simulink model "Adams_HW_Dynamic"  (R2023b)
settings: Solver=VariableStepAuto  StartTime=0.0  StopTime=10.0  RelTol=1e-3
values from neighbouring files (symbols this model uses):
  ddQ1 = x(7)    [Adams_HW1.m]    (also in BSM.m; Correct_new_data.m; MechanicalMechanics_Dynamic.m; MechanicalMechanics_Dynamic_adaptive_BSM.m)
  L1 = x(1)    [Adams_HW1.m]    (also in Adams_HW_DrawGIF.m = current_x(1); Adams_HW_DrawGIF_Y.m = current_x(1); BSM.m; Correct_new_data.m)
  L2 = x(2)    [Adams_HW1.m]    (also in Adams_HW_DrawGIF.m = current_x(2); Adams_HW_DrawGIF_Y.m = current_x(2); BSM.m; Correct_new_data.m)
  L3 = x(3)    [Adams_HW1.m]    (also in Adams_HW_DrawGIF.m = current_x(3); Adams_HW_DrawGIF_Y.m = current_x(3); BSM.m; Correct_new_data.m)
  L4 = x(4)    [Adams_HW1.m]    (also in Adams_HW_DrawGIF.m = current_x(4); Adams_HW_DrawGIF_Y.m = current_x(4); BSM.m; Correct_new_data.m)
  Q1 = x(5)    [Adams_HW1.m]    (also in Adams_HW_DrawGIF.m = current_x(5); Adams_HW_DrawGIF_Y.m = current_x(5); BSM.m; Correct_new_data.m)
  Q2 = Inition(1)    [Adams_HW1.m]    (also in BSM.m = x(8); Correct_new_data.m = x(8); GenerateSimplifiedMechanism.m = x(8); MechanicalMechanics_Dynamic.m = x(8))
  Q3 = x(11)    [Adams_HW1.m]    (also in Adams_HW_DrawGIF.m = current_x(11); Adams_HW_DrawGIF_Y.m = current_x(7); BSM.m; Correct_new_data.m)
settings Model: Creator=Akko  LastModifiedBy=Akko

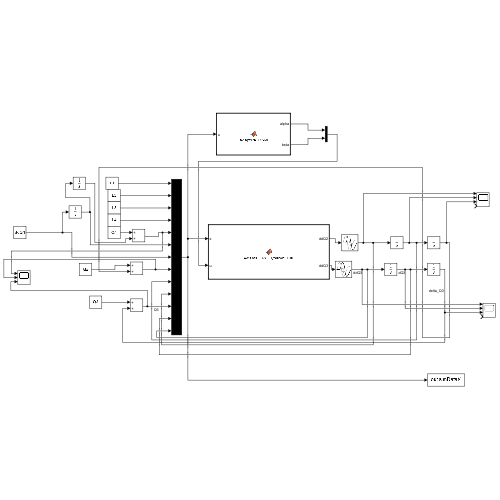
[thumbnail: Simulink's stored preview of the top-level diagram]
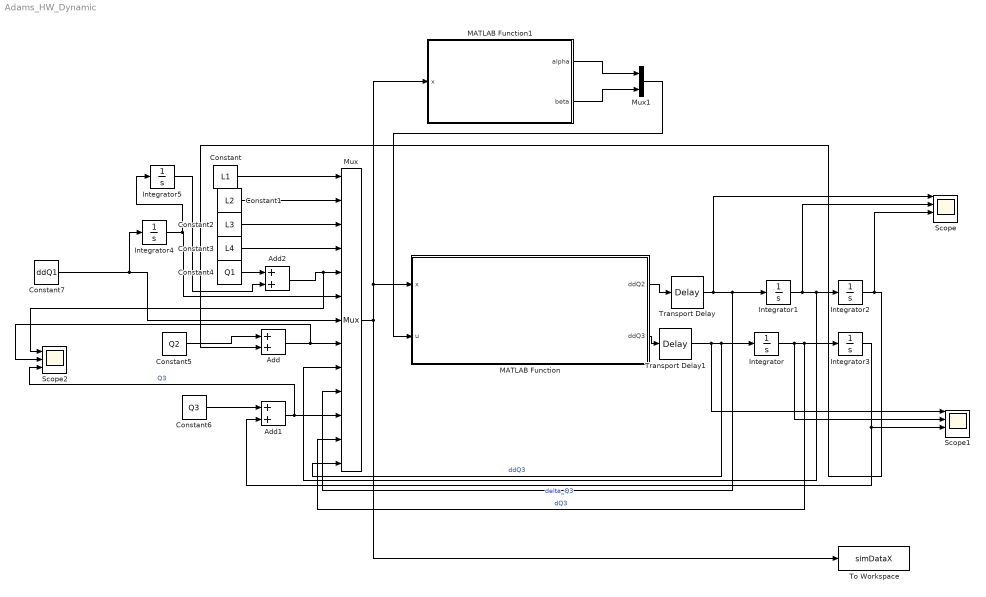
== system Adams_HW_Dynamic ==
  Add : Sum
  Add1 : Sum
  Add2 : Sum
  Constant : Constant  Value=L1
  Constant1 : Constant  Value=L2
  Constant2 : Constant  Value=L3
  Constant3 : Constant  Value=L4
  Constant4 : Constant  Value=Q1
  Constant5 : Constant  Value=Q2
  Constant6 : Constant  Value=Q3
  Constant7 : Constant  Value=ddQ1
  Integrator{,1..5} (6 alike) : Integrator
  MATLAB Function : MATLAB Function  TreatAsAtomicUnit=on
  MATLAB Function1 : MATLAB Function  TreatAsAtomicUnit=on
  Mux : Mux  Inputs=13
  Mux1 : Mux  Inputs=2
  Scope : Scope  NumInputPorts=4
  Scope1 : Scope  NumInputPorts=4
  Scope2 : Scope  NumInputPorts=3
  To Workspace : ToWorkspace  VariableName=simDataX  SampleTime=-1
  Transport Delay : TransportDelay  DelayTime=1e-4
  Transport Delay1 : TransportDelay  DelayTime=1e-4
  wires:
  Mux/1 -> MATLAB Function1/1("x "), MATLAB Function/1(x), To Workspace/1
  Constant/1 -> Mux/1
  Constant1/1 -> Mux/2
  Constant2/1 -> Mux/3
  Constant3/1 -> Mux/4
  MATLAB Function/2(ddQ3) -> Transport Delay1/1
  MATLAB Function/1(ddQ2) -> Transport Delay/1
  Transport Delay1/1 -> Scope1/1, Mux/13, Integrator/1  "ddQ3"
  Transport Delay/1 -> Scope/1, Mux/10, Integrator1/1
  Integrator1/1 -> Scope/2, Mux/9, Integrator2/1
  Integrator/1 -> Scope1/2, Mux/12, Integrator3/1  "dQ3"
  Integrator2/1 -> Scope/3, Add/2
  Constant5/1 -> Add/1
  Add/1 -> Scope2/2, Mux/8
  Add1/1 -> Mux/11, Scope2/3  "Q3"
  Constant6/1 -> Add1/1
  Integrator3/1 -> Scope1/3, Add1/2  "delta_Q3"
  Constant7/1 -> Integrator4/1, Mux/7
  Integrator4/1 -> Integrator5/1, Mux/6
  Add2/1 -> Scope2/1, Mux/5
  Constant4/1 -> Add2/1
  Integrator5/1 -> Add2/2
  MATLAB Function1/1(alpha) -> Mux1/1
  MATLAB Function1/2(beta) -> Mux1/2
  Mux1/1 -> MATLAB Function/2(u)

== matlab function Adams_HW_Dynamic/MATLAB Function ==
  data: x input; ddQ2 output; ddQ3 output; u input
function [ddQ2,ddQ3]=Adams_HW_Dynamic_Cal(x,u)
L1=x(1);L2=x(2);L3=x(3);L4=x(4);
Q1=x(5);dQ1=x(6);ddQ1=x(7);
Q2=x(8);dQ2=x(9);ddQ2=x(10);
Q3=x(11);dQ3=x(12);ddQ3=x(13);
alpha=u(1);beta=u(2);


%BSM法相关定义
%Phi为位置约束列向量
Phi=[ L1*cos(Q1) + L2*cos(Q2) - L3*cos(Q3) - L4;
    L1*sin(Q1) + L2*sin(Q2) - L3*sin(Q3)];

%dot_Phi为速度约束列向量
Jacob=[-L1*sin(Q1),-(L2)*sin(Q2),L3*sin(Q3);
        L1*cos(Q1),(L2)*cos(Q2),-L3*cos(Q3);
];%Q1、Q2、Q3

Phi_t=zeros(2,1);
dot_Phi=Jacob*[dQ1;dQ2;dQ3]+Phi_t;



A_1=[L2*cos(Q2), - L3*cos(Q3);
     L2*sin(Q2) ,- L3*sin(Q3)]*[dQ2^2;dQ3^2];


A_2=[-L2*sin(Q2),  L3*sin(Q3);
      L2*cos(Q2), -L3*cos(Q3)];%*[ddQ2;ddQ3]


b_1=[ L1*sin(Q1); 
     -L1*cos(Q1)]*ddQ1;
b_2=[L1*cos(Q1);L1*sin(Q1)]*((dQ1)^2);

b=((b_1+b_2)-A_1)-(2*alpha*dot_Phi+(beta^2)*Phi);

if abs(det(A_2)) < 1e-6
    % 如果矩阵接近奇异，使用伪逆 (pinv) 或者输出 0 防止报错
    y = pinv(A_2) * b; 
else
    y = A_2\b;
end

ddQ2=y(1);
ddQ3=y(2);
end

== matlab function Adams_HW_Dynamic/MATLAB Function1 ==
  data: x input size=13; alpha output; beta output
function [alpha,beta] = adaptive_BSM(x)
L1=x(1);L2=x(2);L3=x(3);L4=x(4);
Q1=x(5);dQ1=x(6);ddQ1=x(7);
Q2=x(8);dQ2=x(9);ddQ2=x(10);
Q3=x(11);dQ3=x(12);ddQ3=x(13);

    n = 2; % 默认约束方程个数
%BSM法相关定义
%Phi为位置约束列向量
Phi=[ L1*cos(Q1) + L2*cos(Q2) - L3*cos(Q3) - L4;
    L1*sin(Q1) + L2*sin(Q2) - L3*sin(Q3)];

%dot_Phi为速度约束列向量
Jacob=[-L1*sin(Q1),-(L2)*sin(Q2),L3*sin(Q3);
        L1*cos(Q1),(L2)*cos(Q2),-L3*cos(Q3);
];%Q1、Q2、Q3

Phi_t=zeros(2,1);
dot_Phi=Jacob*[dQ1;dQ2;dQ3]+Phi_t;


% 2. 计算模长，加上 eps 防止 log(0)
norm_Phi = sqrt(Phi'*Phi/n);
norm_dotPhi = sqrt(dot_Phi'*dot_Phi/n);

% 使用 log10 替换 lg，并加入 eps 防止负无穷
err_Phi = log10(norm_Phi +eps); 
err_dotPhi = log10(norm_dotPhi +eps); 

%定义计算误差、乘法函数
err=1;%定步长算法

% 定义分段函数
ec = @(z) (z >= -6) * 10 + (z <= -16) * 0 + ...
          (z > -16 & z < -6) .* (16 + z);

y=@(z) 10*err*ec(z);

%计算算子
alpha=y(err_dotPhi);
beta=y(err_Phi);
%做数据保护
alpha = min(max(alpha,0),100); beta = min(max(beta,0),100);
end
